simulink model "Tumbller_STR"  (R2019a)
settings: Solver=ode45  StartTime=t0  StopTime=tend  MaxStep=maxstep  RelTol=tol  AbsTol=tol
values from neighbouring files (symbols this model uses):
  eq = [0; 0; 0; 0]    [Sim_STR.m]
  K0 = lqr(A_sys, B_sys, Q, R)    [Sim_STR.m]
  lambda = 0.995    [Sim_STR.m]
  P0 = 1e8 * eye(n_theta)    [Sim_STR.m]
  Q = 1000*eye(4)    [Sim_STR.m]
  R = 1    [Sim_STR.m]
  T = 0.015    [Sim_STR.m]
  theta0 = [-3.3899 -0.9880 -4.4196 -0.0958 0.4707 3.7728].'    [Sim_STR.m]
  update_ctlr = 1    [Sim_STR.m]
  z0 = x0    [Sim_STR.m]
undefined symbols (not defined in the file or in its folder): motorparams, params
libraries: simulink x1, dspstat3 x1
settings Model: Creator=bednarse  LastModifiedBy=bednarse

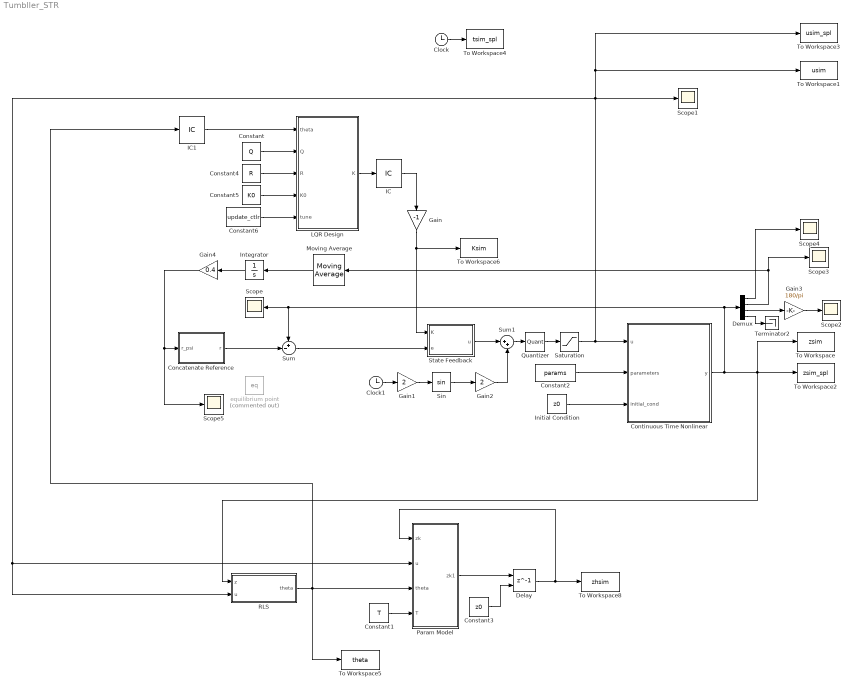
== system Tumbller_STR ==
  Clock : Clock
  Clock1 : Clock
  Concatenate Reference : MATLAB Function  TreatAsAtomicUnit=on
  Constant : Constant  Value=Q
  Constant1 : Constant  Value=T
  Constant2 : Constant  Value=params
  Constant3 : Constant  Value=z0
  Constant4 : Constant  Value=R
  Constant5 : Constant  Value=K0  VectorParams1D=off
  Constant6 : Constant  Value=update_ctlr
  Continuous Time Nonlinear : Subsystem
  Delay : Delay  DelayLength=1  InitialConditionSource=Input port
      settings: InputPortMap=u0,p4
  Demux : Demux
  Gain : Gain  Gain=-1
  Gain1 : Gain  Gain=2
  Gain2 : Gain  Gain=2
  Gain3 : Gain  Gain=180/pi
  Gain4 : Gain  Gain=0.4
  IC : InitialCondition  Value=K0
  IC1 : InitialCondition  Value=theta0
  Initial Condition : Constant  Value=z0
  Integrator : Integrator
  LQR Design : MATLAB Function  TreatAsAtomicUnit=on  SystemSampleTime=T
  Moving Average : dspstat3/Moving Average  Method=Sliding window  ForgettingFactorPort=off  SpecifyWindowLength=on  WindowLength=50  ForgettingFactor=0.9  SimulateUsing=Interpreted execution
  Param Model : MATLAB Function  TreatAsAtomicUnit=on  SystemSampleTime=T
  Quantizer : Quantizer  QuantizationInterval=8/255
  RLS : Subsystem
  Saturation : Saturate  UpperLimit=8  LowerLimit=-8
  Scope{,1..5} (6 alike) : Scope
  Sin : Trigonometry
  State Feedback : MATLAB Function  TreatAsAtomicUnit=on
  Sum : Sum  Inputs=+-|
  Sum1 : Sum  Inputs=|++
  Terminator2 : Terminator
  To Workspace : ToWorkspace  VariableName=zsim  SampleTime=-1
  To Workspace1 : ToWorkspace  VariableName=usim  SampleTime=-1
  To Workspace2 : ToWorkspace  VariableName=zsim_spl  SampleTime=T
  To Workspace3 : ToWorkspace  VariableName=usim_spl  SampleTime=T
  To Workspace4 : ToWorkspace  VariableName=tsim_spl  SampleTime=T
  To Workspace5 : ToWorkspace  VariableName=theta  SampleTime=T
  To Workspace6 : ToWorkspace  VariableName=Ksim  SaveFormat=Timeseries  SampleTime=T
  To Workspace8 : ToWorkspace  VariableName=zhsim  SampleTime=T
  equilibrium point : Constant  Commented=on  Value=eq
  wires:
  Clock/1 -> To Workspace4/1
  Param Model/1(zk1) -> Delay/1
  Constant1/1 -> Param Model/4(T)
  Constant3/1 -> Delay/2
  Delay/1 -> Param Model/1(zk), To Workspace8/1
  RLS/1(theta) -> IC1/1, Param Model/3(theta), To Workspace5/1
  Constant2/1 -> Continuous Time Nonlinear/2(parameters)
  Continuous Time Nonlinear/1(y) -> To Workspace/1, RLS/1(z), To Workspace2/1, Demux/1, Scope/1, Sum/1
  Initial Condition/1 -> Continuous Time Nonlinear/3(initial_cond)
  Clock1/1 -> Gain1/1
  Gain1/1 -> Sin/1
  Sin/1 -> Gain2/1
  Sum1/1 -> Quantizer/1
  Gain2/1 -> Sum1/2
  Demux/4 -> Terminator2/1
  Gain3/1 -> Scope2/1
  Saturation/1 -> Param Model/2(u), RLS/2(u), To Workspace3/1, To Workspace1/1, Scope1/1, Continuous Time Nonlinear/1(u)
  Constant5/1 -> LQR Design/4(K0)
  Constant6/1 -> LQR Design/5(tune)
  Constant4/1 -> LQR Design/3(R)
  Constant/1 -> LQR Design/2(Q)
  LQR Design/1(K) -> IC/1
  IC1/1 -> LQR Design/1(theta)
  State Feedback/1(u) -> Sum1/1
  Sum/1 -> State Feedback/2(e)
  IC/1 -> Gain/1
  Gain/1 -> To Workspace6/1, State Feedback/1(K)
  Demux/1 -> Scope4/1
  Demux/3 -> Gain3/1
  Demux/2 -> Moving Average/1, Scope3/1
  Moving Average/1 -> Integrator/1
  Integrator/1 -> Gain4/1
  Gain4/1 -> Scope5/1, Concatenate Reference/1(r_psi)
  Concatenate Reference/1(r) -> Sum/2
  Quantizer/1 -> Saturation/1

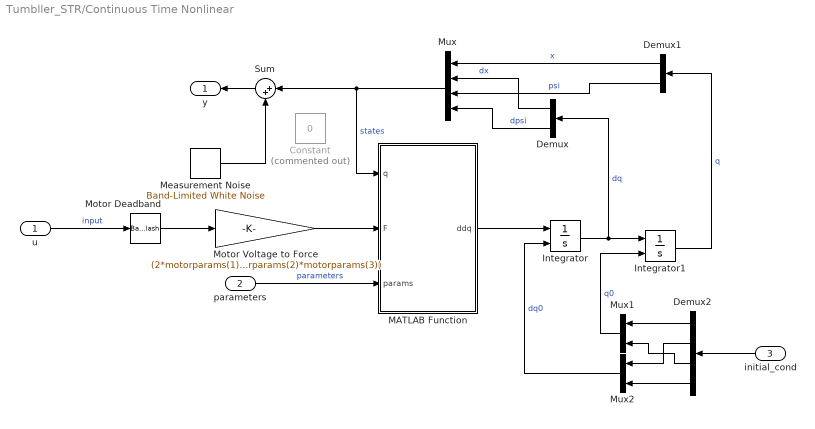
== system Tumbller_STR/Continuous Time Nonlinear ==
  u : Inport
  parameters : Inport  Port=2
  initial_cond : Inport  Port=3
  Constant : Constant  Commented=on  Value=0
  Demux : Demux  Outputs=2
  Demux1 : Demux  Outputs=2
  Demux2 : Demux
  Integrator : Integrator  InitialConditionSource=external
  Integrator1 : Integrator  InitialConditionSource=external
  MATLAB Function : MATLAB Function  TreatAsAtomicUnit=on
  Measurement Noise : simulink/Sources/Band-Limited White Noise  Cov=[1e-6 1e-6 1e-6 1e-6]  Ts=0.01  seed=[23341]
  Motor Deadband : Backlash
  Motor Voltage to Force : Gain  Gain=(2*motorparams(1))/(motorparams(2)*motorparams(3))
  Mux : Mux
  Mux1 : Mux  Inputs=2
  Mux2 : Mux  Inputs=2
  Sum : Sum  Inputs=|++
  y : Outport  VectorParamsAs1DForOutWhenUnconnected=on
  wires:
  Demux1/1 -> Mux/1  "x"
  Integrator/1 -> Demux/1, Integrator1/1  "dq"
  Integrator1/1 -> Demux1/1  "q"
  Demux2/1 -> Mux1/1
  Mux1/1 -> Integrator1/2  "q0"
  Demux2/4 -> Mux2/2
  Demux1/2 -> Mux/3  "psi"
  Demux/2 -> Mux/4  "dpsi"
  MATLAB Function/1(ddq) -> Integrator/1
  Mux2/1 -> Integrator/2  "dq0"
  Demux2/2 -> Mux2/1
  Demux2/3 -> Mux1/2
  Demux/1 -> Mux/2  "dx"
  initial_cond/1 -> Demux2/1
  Mux/1 -> Sum/1, MATLAB Function/1(q)  "states"
  parameters/1 -> MATLAB Function/3(params)  "parameters"
  Sum/1 -> y/1
  Motor Voltage to Force/1 -> MATLAB Function/2(F)
  u/1 -> Motor Deadband/1  "input"
  Motor Deadband/1 -> Motor Voltage to Force/1
  Measurement Noise/1 -> Sum/2

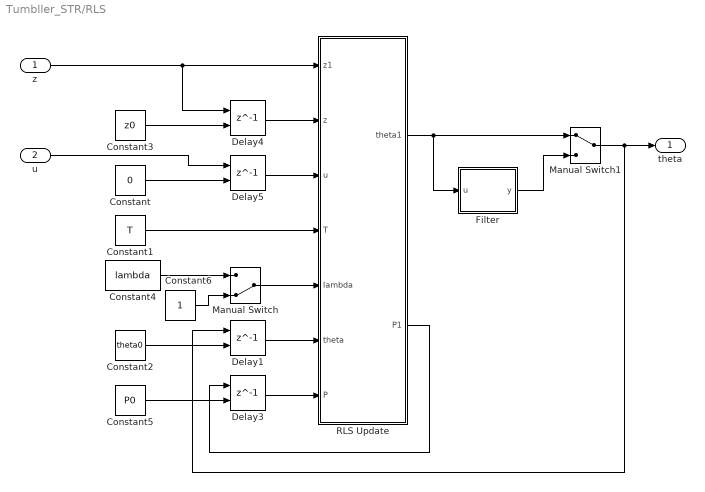
== system Tumbller_STR/RLS ==
  z : Inport
  u : Inport  Port=2
  Constant : Constant  Value=0
  Constant1 : Constant  Value=T
  Constant2 : Constant  Value=theta0
  Constant3 : Constant  Value=z0
  Constant4 : Constant  Value=lambda
  Constant5 : Constant  Value=P0
  Constant6 : Constant
  Delay{1,3..5} (4 alike) : Delay  DelayLength=1  InitialConditionSource=Input port
      settings: InputPortMap=u0,p4
  Filter : Subsystem
  Manual Switch : ManualSwitch  CurrentSetting=0
  Manual Switch1 : ManualSwitch
  RLS Update : MATLAB Function  TreatAsAtomicUnit=on  SystemSampleTime=T
  theta : Outport
  wires:
  Constant/1 -> Delay5/2
  Constant3/1 -> Delay4/2
  Constant5/1 -> Delay3/2
  Constant1/1 -> RLS Update/4(T)
  Constant2/1 -> Delay1/2
  Delay5/1 -> RLS Update/3(u)
  Delay4/1 -> RLS Update/2(z)
  Delay3/1 -> RLS Update/7(P)
  Delay1/1 -> RLS Update/6(theta)
  RLS Update/2(P1) -> Delay3/1
  u/1 -> Delay5/1
  z/1 -> Delay4/1, RLS Update/1(z1)
  Manual Switch/1 -> RLS Update/5(lambda)
  Constant6/1 -> Manual Switch/2
  Constant4/1 -> Manual Switch/1
  Manual Switch1/1 -> Delay1/1, theta/1
  RLS Update/1(theta1) -> Manual Switch1/1, Filter/1(u)
  Filter/1(y) -> Manual Switch1/2

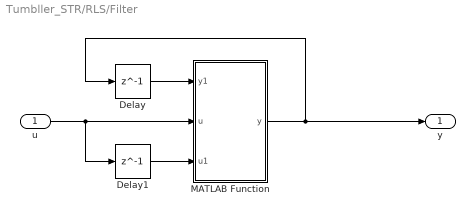
== system Tumbller_STR/RLS/Filter ==
  u : Inport
  Delay : Delay  DelayLength=1  InitialCondition=theta0
  Delay1 : Delay  DelayLength=1  InitialCondition=theta0
  MATLAB Function : MATLAB Function  TreatAsAtomicUnit=on  SystemSampleTime=T
  y : Outport
  wires:
  u/1 -> Delay1/1, MATLAB Function/2(u)
  Delay/1 -> MATLAB Function/1(y1)
  Delay1/1 -> MATLAB Function/3(u1)
  MATLAB Function/1(y) -> Delay/1, y/1

== matlab function Tumbller_STR/LQR Design ==
  data: theta input; K output size=[1 4]; Q input; R input; K0 input; tune input
function K = design_ctlr(theta, Q, R, K0, tune)

K = [0 0 0 0];
coder.extrinsic('lqr'); 

if(tune)
    A = [0 1 0 0; ...
    0 theta(1:2).' 0; ...
    0 0 0 1; ...
    0 theta(3:4).' 0];
    B = [0 theta(5) 0 theta(6)].';
    K = lqr(A, B, Q, R);
else
    K = K0;
end

== matlab function Tumbller_STR/Continuous Time Nonlinear/MATLAB Function ==
  data: q input size=[1 4]; ddq output size=[2 1]; F input; params input size=[1 11]
function ddq = fcn(q, F, params)
ddq = offsetdyn_fun([q(1), q(2), q(3), q(4)], F, params);

== matlab function Tumbller_STR/Param Model ==
  data: zk input; u input; zk1 output size=4; theta input; T input
function zk1 = fcn(zk, u, theta, T)

A = [0 1 0 0; ...
    0 theta(1:2).' 0; ...
    0 0 0 1; ...
    0 theta(3:4).' 0];
B = [0 theta(5) 0 theta(6)].';

Ad = eye(4) + T * A;
Bd = T * B;

zk1 = Ad*zk + Bd*u;

== matlab function Tumbller_STR/RLS/Filter/MATLAB Function ==
  data: y1 input; u input; y output; u1 input
function y = lpf(y1, u, u1)

% b1 = 0.04837;
% b0 = 0.04679;
% a0 = -0.9048;

% b1 = 0.9;
% b0 = 0.09995;
% a0 = -4.54e-5;

b1 = 0;
b0 = 1;
a0 = -4.54e-5;

y = b1*u + b0*u1 - a0*y1;

== matlab function Tumbller_STR/RLS/RLS Update ==
  data: z1 input; z input; u input; T input; lambda input; theta input; P input; theta1 output size=6; P1 output size=[6 6]
function[theta1, P1] =  msd2_rls(z1, z, u, T, lambda, theta, P)
    [phi, delta] = linParamFunc(z, u, T);
    
    KN = P * phi / (lambda * eye(4) + phi.' * P * phi);
    theta1 = theta + KN * (z1 - delta - phi.' * theta);
    P1 = (eye(6) - KN * phi.') * P / lambda;
end


function[phi, delta] = linParamFunc(z, u, T)
    phi = zeros(6, 4);
    phi(1:2, 2) = T * z(2:3);
    phi(5, 2) = T * u;
    phi(3:4, 4) = T * z(2:3);
    phi(6, 4) = T * u;
    
    delta = [z(1)+T*z(2); ...
                    z(2); ...
             z(3)+T*z(4); ...
                    z(4)];
end

== matlab function Tumbller_STR/State Feedback ==
  data: K input; u output; e input
function u = ctlr(K, e)

u = K.' * e;

== matlab function Tumbller_STR/Concatenate Reference ==
  data: r_psi input; r output
function r = fcn(r_psi)

r = [0; 0; r_psi; 0];
